simulink model "ROPOD_dynamic_model_sim_Wheel_Input"  (R2016b)
settings: Solver=FixedStepAuto  StartTime=0.0  StopTime=timesim(end)  FixedStep=Ts  MaxStep=1e-3  RelTol=1e-3
values from neighbouring files (symbols this model uses):
  ropod_dynmodel_pv = struct2array(ropod_dynmodel_param)    [set_ropod_configparams_sim.m]
(part 3 of 4)

== matlab function ROPOD_dynamic_model_sim_Wheel_Input/Feedback Linearization/M_matrix_c ==
  data: ropod_dynmodel_pv input; M output; qin input
function M   = M_matrix( ropod_dynmodel_pv, qin)
%ROPOD_JACOBIAN Summary of this function goes here
%   Detailed explanation goes here


r_w     = ropod_dynmodel_pv(1);
s_w     = ropod_dynmodel_pv(2);
d_w     = ropod_dynmodel_pv(3);
l_CW    = ropod_dynmodel_pv(4);

Mr = ropod_dynmodel_pv(5);
Ir = ropod_dynmodel_pv(6);
Mwma = ropod_dynmodel_pv(7);
Iwma = ropod_dynmodel_pv(8);
Mwca = ropod_dynmodel_pv(9);
Iwca = ropod_dynmodel_pv(10);
Mw   = ropod_dynmodel_pv(11);
Iwz  = ropod_dynmodel_pv(12);
Iwp  = ropod_dynmodel_pv(13);


% Map state vector to the corresponfing variables
xc      = qin(1);
yc      = qin(2);
theta   = qin(3);
delta   = qin(4:7);
varphi  = qin(8:15);

delta1 = delta(1);
delta2 = delta(2);
delta3 = delta(3);
delta4 = delta(4);

M = [
[ (4*Iwp*d_w^2 + 8*Iwca*r_w^2 + 8*Iwma*r_w^2 + 16*Iwz*r_w^2 + 16*Iwp*s_w^2 + 4*Mw*d_w^2*r_w^2 + 4*Mr*r_w^2*s_w^2 + 16*Mw*r_w^2*s_w^2 + 10*Mwca*r_w^2*s_w^2 + 8*Mwma*r_w^2*s_w^2 - Iwp*d_w^2*cos(2*delta1 + 2*theta) - Iwp*d_w^2*cos(2*delta2 + 2*theta) - Iwp*d_w^2*cos(2*delta3 + 2*theta) - Iwp*d_w^2*cos(2*delta4 + 2*theta) - 2*Iwca*r_w^2*cos(2*delta1 + 2*theta) - 2*Iwca*r_w^2*cos(2*delta2 + 2*theta) - 2*Iwca*r_w^2*cos(2*delta3 + 2*theta) - 2*Iwca*r_w^2*cos(2*delta4 + 2*theta) - 2*Iwma*r_w^2*cos(2*delta1 + 2*theta) - 2*Iwma*r_w^2*cos(2*delta2 + 2*theta) - 2*Iwma*r_w^2*cos(2*delta3 + 2*theta) - 2*Iwma*r_w^2*cos(2*delta4 + 2*theta) - 4*Iwz*r_w^2*cos(2*delta1 + 2*theta) - 4*Iwz*r_w^2*cos(2*delta2 + 2*theta) - 4*Iwz*r_w^2*cos(2*delta3 + 2*theta) - 4*Iwz*r_w^2*cos(2*delta4 + 2*theta) + 4*Iwp*s_w^2*cos(2*delta1 + 2*theta) + 4*Iwp*s_w^2*cos(2*delta2 + 2*theta) + 4*Iwp*s_w^2*cos(2*delta3 + 2*theta) + 4*Iwp*s_w^2*cos(2*delta4 + 2*theta) - Mw*d_w^2*r_w^2*cos(2*delta1 + 2*theta) - Mw*d_w^2*r_w^2*cos(2*delta2 + 2*theta) - Mw*d_w^2*r_w^2*cos(2*delta3 + 2*theta) - Mw*d_w^2*r_w^2*cos(2*delta4 + 2*theta) + 4*Mw*r_w^2*s_w^2*cos(2*delta1 + 2*theta) + 4*Mw*r_w^2*s_w^2*cos(2*delta2 + 2*theta) + 4*Mw*r_w^2*s_w^2*cos(2*delta3 + 2*theta) + 4*Mw*r_w^2*s_w^2*cos(2*delta4 + 2*theta) + (3*Mwca*r_w^2*s_w^2*cos(2*delta1 + 2*theta))/2 + (3*Mwca*r_w^2*s_w^2*cos(2*delta2 + 2*theta))/2 + (3*Mwca*r_w^2*s_w^2*cos(2*delta3 + 2*theta))/2 + (3*Mwca*r_w^2*s_w^2*cos(2*delta4 + 2*theta))/2 + 2*Mwma*r_w^2*s_w^2*cos(2*delta1 + 2*theta) + 2*Mwma*r_w^2*s_w^2*cos(2*delta2 + 2*theta) + 2*Mwma*r_w^2*s_w^2*cos(2*delta3 + 2*theta) + 2*Mwma*r_w^2*s_w^2*cos(2*delta4 + 2*theta))/(4*r_w^2*s_w^2),                                                                                                                                                                                                                                                                                                                                                                                                                                                                                                                                                                                                                                                                                                                                                                                                                                                                                                                                                                                                                                                                                                                                                                                                                                                                                                                                                                                                                                             -((sin(2*delta1 + 2*theta) + sin(2*delta2 + 2*theta) + sin(2*delta3 + 2*theta) + sin(2*delta4 + 2*theta))*(Iwp*d_w^2 + 2*Iwca*r_w^2 + 2*Iwma*r_w^2 + 4*Iwz*r_w^2 - 4*Iwp*s_w^2 + Mw*d_w^2*r_w^2 - 4*Mw*r_w^2*s_w^2 - (3*Mwca*r_w^2*s_w^2)/2 - 2*Mwma*r_w^2*s_w^2))/(4*r_w^2*s_w^2),                                                                                                                                                                                                                                                                                                                                                                                                                                                                                                                                                                                                                                                                                                                                                                                                                                                                                                                                                                                                                                                                                                                                                                                                                                                                                                                                                                   (2^(1/2)*l_CW*(cos(2*delta1 + theta + pi/4) - cos(2*delta3 + theta + pi/4) - sin(2*delta2 + theta + pi/4) + sin(2*delta4 + theta + pi/4))*(2*Iwp*d_w^2 + 4*Iwca*r_w^2 + 4*Iwma*r_w^2 + 8*Iwz*r_w^2 - 8*Iwp*s_w^2 + 2*Mw*d_w^2*r_w^2 - 8*Mw*r_w^2*s_w^2 - 3*Mwca*r_w^2*s_w^2 - 4*Mwma*r_w^2*s_w^2))/(8*r_w^2*s_w^2)];
[                                                                                                                                                                                                                                                                                                                                                                                                                                                                                                                                                                                                                                                                                                                                                                                                                                                                                                                                                                                                                                                                                                                                                                                                                                                                                                                                                                                                                                             -((sin(2*delta1 + 2*theta) + sin(2*delta2 + 2*theta) + sin(2*delta3 + 2*theta) + sin(2*delta4 + 2*theta))*(Iwp*d_w^2 + 2*Iwca*r_w^2 + 2*Iwma*r_w^2 + 4*Iwz*r_w^2 - 4*Iwp*s_w^2 + Mw*d_w^2*r_w^2 - 4*Mw*r_w^2*s_w^2 - (3*Mwca*r_w^2*s_w^2)/2 - 2*Mwma*r_w^2*s_w^2))/(4*r_w^2*s_w^2), (4*Iwp*d_w^2 + 8*Iwca*r_w^2 + 8*Iwma*r_w^2 + 16*Iwz*r_w^2 + 16*Iwp*s_w^2 + 4*Mw*d_w^2*r_w^2 + 4*Mr*r_w^2*s_w^2 + 16*Mw*r_w^2*s_w^2 + 10*Mwca*r_w^2*s_w^2 + 8*Mwma*r_w^2*s_w^2 + Iwp*d_w^2*cos(2*delta1 + 2*theta) + Iwp*d_w^2*cos(2*delta2 + 2*theta) + Iwp*d_w^2*cos(2*delta3 + 2*theta) + Iwp*d_w^2*cos(2*delta4 + 2*theta) + 2*Iwca*r_w^2*cos(2*delta1 + 2*theta) + 2*Iwca*r_w^2*cos(2*delta2 + 2*theta) + 2*Iwca*r_w^2*cos(2*delta3 + 2*theta) + 2*Iwca*r_w^2*cos(2*delta4 + 2*theta) + 2*Iwma*r_w^2*cos(2*delta1 + 2*theta) + 2*Iwma*r_w^2*cos(2*delta2 + 2*theta) + 2*Iwma*r_w^2*cos(2*delta3 + 2*theta) + 2*Iwma*r_w^2*cos(2*delta4 + 2*theta) + 4*Iwz*r_w^2*cos(2*delta1 + 2*theta) + 4*Iwz*r_w^2*cos(2*delta2 + 2*theta) + 4*Iwz*r_w^2*cos(2*delta3 + 2*theta) + 4*Iwz*r_w^2*cos(2*delta4 + 2*theta) - 4*Iwp*s_w^2*cos(2*delta1 + 2*theta) - 4*Iwp*s_w^2*cos(2*delta2 + 2*theta) - 4*Iwp*s_w^2*cos(2*delta3 + 2*theta) - 4*Iwp*s_w^2*cos(2*delta4 + 2*theta) + Mw*d_w^2*r_w^2*cos(2*delta1 + 2*theta) + Mw*d_w^2*r_w^2*cos(2*delta2 + 2*theta) + Mw*d_w^2*r_w^2*cos(2*delta3 + 2*theta) + Mw*d_w^2*r_w^2*cos(2*delta4 + 2*theta) - 4*Mw*r_w^2*s_w^2*cos(2*delta1 + 2*theta) - 4*Mw*r_w^2*s_w^2*cos(2*delta2 + 2*theta) - 4*Mw*r_w^2*s_w^2*cos(2*delta3 + 2*theta) - 4*Mw*r_w^2*s_w^2*cos(2*delta4 + 2*theta) - (3*Mwca*r_w^2*s_w^2*cos(2*delta1 + 2*theta))/2 - (3*Mwca*r_w^2*s_w^2*cos(2*delta2 + 2*theta))/2 - (3*Mwca*r_w^2*s_w^2*cos(2*delta3 + 2*theta))/2 - (3*Mwca*r_w^2*s_w^2*cos(2*delta4 + 2*theta))/2 - 2*Mwma*r_w^2*s_w^2*cos(2*delta1 + 2*theta) - 2*Mwma*r_w^2*s_w^2*cos(2*delta2 + 2*theta) - 2*Mwma*r_w^2*s_w^2*cos(2*delta3 + 2*theta) - 2*Mwma*r_w^2*s_w^2*cos(2*delta4 + 2*theta))/(4*r_w^2*s_w^2),                                                                                                                                                                                                                                                                                                                                                                                                                                                                                                                                                                                                                                                                                                                                                                                                                                                                                                                                                                                                                                                                                                                                                                                                                                                                                                                                                                   (2^(1/2)*l_CW*(cos(2*delta2 + theta + pi/4) - cos(2*delta4 + theta + pi/4) + sin(2*delta1 + theta + pi/4) - sin(2*delta3 + theta + pi/4))*(2*Iwp*d_w^2 + 4*Iwca*r_w^2 + 4*Iwma*r_w^2 + 8*Iwz*r_w^2 - 8*Iwp*s_w^2 + 2*Mw*d_w^2*r_w^2 - 8*Mw*r_w^2*s_w^2 - 3*Mwca*r_w^2*s_w^2 - 4*Mwma*r_w^2*s_w^2))/(8*r_w^2*s_w^2)];
[                                                                                                                                                                                                                                                                                                                                                                                                                                                                                                                                                                                                                                                                                                                                                                                                                                                                                                                                                                                                                                                                                                                                                                                                                                                                                                                                                                                                             (2^(1/2)*l_CW*(cos(2*delta1 + theta + pi/4) - cos(2*delta3 + theta + pi/4) - sin(2*delta2 + theta + pi/4) + sin(2*delta4 + theta + pi/4))*(2*Iwp*d_w^2 + 4*Iwca*r_w^2 + 4*Iwma*r_w^2 + 8*Iwz*r_w^2 - 8*Iwp*s_w^2 + 2*Mw*d_w^2*r_w^2 - 8*Mw*r_w^2*s_w^2 - 3*Mwca*r_w^2*s_w^2 - 4*Mwma*r_w^2*s_w^2))/(8*r_w^2*s_w^2),                                                                                                                                                                                                                                                                                                                                                                                                                                                                                                                                                                                                                                                                                                                                                                                                                                                                                                                                                                                                                                                                                                                                                                                                                                                                                                                                                                                                             (2^(1/2)*l_CW*(cos(2*delta2 + theta + pi/4) - cos(2*delta4 + theta + pi/4) + sin(2*delta1 + theta + pi/4) - sin(2*delta3 + theta + pi/4))*(2*Iwp*d_w^2 + 4*Iwca*r_w^2 + 4*Iwma*r_w^2 + 8*Iwz*r_w^2 - 8*Iwp*s_w^2 + 2*Mw*d_w^2*r_w^2 - 8*Mw*r_w^2*s_w^2 - 3*Mwca*r_w^2*s_w^2 - 4*Mwma*r_w^2*s_w^2))/(8*r_w^2*s_w^2), (8*Iwp*d_w^2*l_CW^2 + 16*Iwca*l_CW^2*r_w^2 + 16*Iwma*l_CW^2*r_w^2 + 32*Iwz*l_CW^2*r_w^2 + 32*Iwp*l_CW^2*s_w^2 + 4*Ir*r_w^2*s_w^2 + 8*Mw*d_w^2*l_CW^2*r_w^2 + 32*Mw*l_CW^2*r_w^2*s_w^2 + 20*Mwca*l_CW^2*r_w^2*s_w^2 + 16*Mwma*l_CW^2*r_w^2*s_w^2 + 2*Iwp*d_w^2*l_CW^2*sin(2*delta1) - 2*Iwp*d_w^2*l_CW^2*sin(2*delta2) + 2*Iwp*d_w^2*l_CW^2*sin(2*delta3) - 2*Iwp*d_w^2*l_CW^2*sin(2*delta4) + 4*Iwca*l_CW^2*r_w^2*sin(2*delta1) - 4*Iwca*l_CW^2*r_w^2*sin(2*delta2) + 4*Iwca*l_CW^2*r_w^2*sin(2*delta3) - 4*Iwca*l_CW^2*r_w^2*sin(2*delta4) + 4*Iwma*l_CW^2*r_w^2*sin(2*delta1) - 4*Iwma*l_CW^2*r_w^2*sin(2*delta2) + 4*Iwma*l_CW^2*r_w^2*sin(2*delta3) - 4*Iwma*l_CW^2*r_w^2*sin(2*delta4) + 8*Iwz*l_CW^2*r_w^2*sin(2*delta1) - 8*Iwz*l_CW^2*r_w^2*sin(2*delta2) + 8*Iwz*l_CW^2*r_w^2*sin(2*delta3) - 8*Iwz*l_CW^2*r_w^2*sin(2*delta4) - 8*Iwp*l_CW^2*s_w^2*sin(2*delta1) + 8*Iwp*l_CW^2*s_w^2*sin(2*delta2) - 8*Iwp*l_CW^2*s_w^2*sin(2*delta3) + 8*Iwp*l_CW^2*s_w^2*sin(2*delta4) + 2*Mw*d_w^2*l_CW^2*r_w^2*sin(2*delta1) - 2*Mw*d_w^2*l_CW^2*r_w^2*sin(2*delta2) + 2*Mw*d_w^2*l_CW^2*r_w^2*sin(2*delta3) - 2*Mw*d_w^2*l_CW^2*r_w^2*sin(2*delta4) - 8*Mw*l_CW^2*r_w^2*s_w^2*sin(2*delta1) + 8*Mw*l_CW^2*r_w^2*s_w^2*sin(2*delta2) - 8*Mw*l_CW^2*r_w^2*s_w^2*sin(2*delta3) + 8*Mw*l_CW^2*r_w^2*s_w^2*sin(2*delta4) - 3*Mwca*l_CW^2*r_w^2*s_w^2*sin(2*delta1) + 3*Mwca*l_CW^2*r_w^2*s_w^2*sin(2*delta2) - 3*Mwca*l_CW^2*r_w^2*s_w^2*sin(2*delta3) + 3*Mwca*l_CW^2*r_w^2*s_w^2*sin(2*delta4) - 4*Mwma*l_CW^2*r_w^2*s_w^2*sin(2*delta1) + 4*Mwma*l_CW^2*r_w^2*s_w^2*sin(2*delta2) - 4*Mwma*l_CW^2*r_w^2*s_w^2*sin(2*delta3) + 4*Mwma*l_CW^2*r_w^2*s_w^2*sin(2*delta4))/(4*r_w^2*s_w^2)];
 ];


end
